simulink model "barcatet_slow_faraHold5cazuri"  (R2021a)
settings: Solver=ode8  StartTime=0.0  StopTime=inf  FixedStep=0.1  RelTol=1e-3
undefined symbols (not defined in the file): carma, distantaLimDr, distantaLimFata, distantaLimSt, motDr, motSt, V0
libraries: simulink x5, arduinolib x3, arduinosensorlib x3
settings Model: SILPILModeSetting=veronly  ExtModeTrigDuration=2  Creator=CANDRONE  LastModifiedBy=Aspire 5
settings OptimizationCC: EnhancedBackFolding=on  PassReuseOutputArgsAs=Individual arguments  ZeroExternalMemoryAtStartup=off  ZeroInternalMemoryAtStartup=off  MaxStackSize=64  OptimizeBlockOrder=speed  DifferentSizesBufferReuse=on  OptimizationCustomize=off  EfficientTunableParamExpr=on
settings DebuggingCC: ParameterTunabilityLossMsg=error
settings HardwareCC: ProdBitPerInt=16  ProdBitPerPointer=16  ProdBitPerSizeT=16  ProdBitPerPtrDiffT=16  ProdLargestAtomicFloat=None  ProdWordSize=8  ProdHWDeviceType=Atmel->AVR
settings SFSimCC: MATLABDynamicMemAlloc=off
settings RTWCC: SystemTargetFile=ert.tlc  HardwareBoard=Arduino Mega 2560  TemplateMakefile=ert_default_tmf  Toolchain=Arduino AVR
settings CodeAppCC: ForceParamTrailComments=on  IgnoreCustomStorageClasses=off  OperatorAnnotations=on  SimulinkDataObjDesc=on  SFDataObjDesc=on  InsertBlockDesc=on
settings ERTTargetCC: SupportContinuousTime=on  SupportVariableSizeSignals=on  ExtModeStaticAllocSize=2048

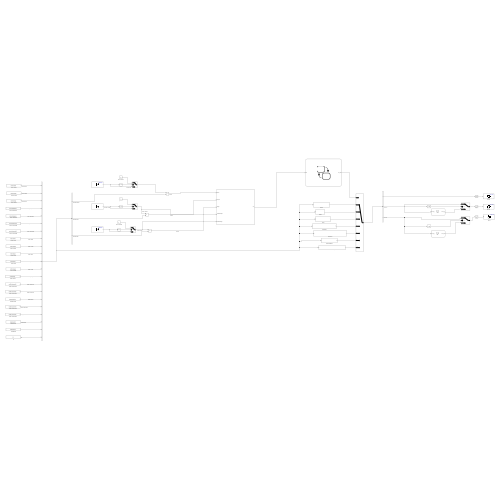
[thumbnail: Simulink's stored preview of the top-level diagram]
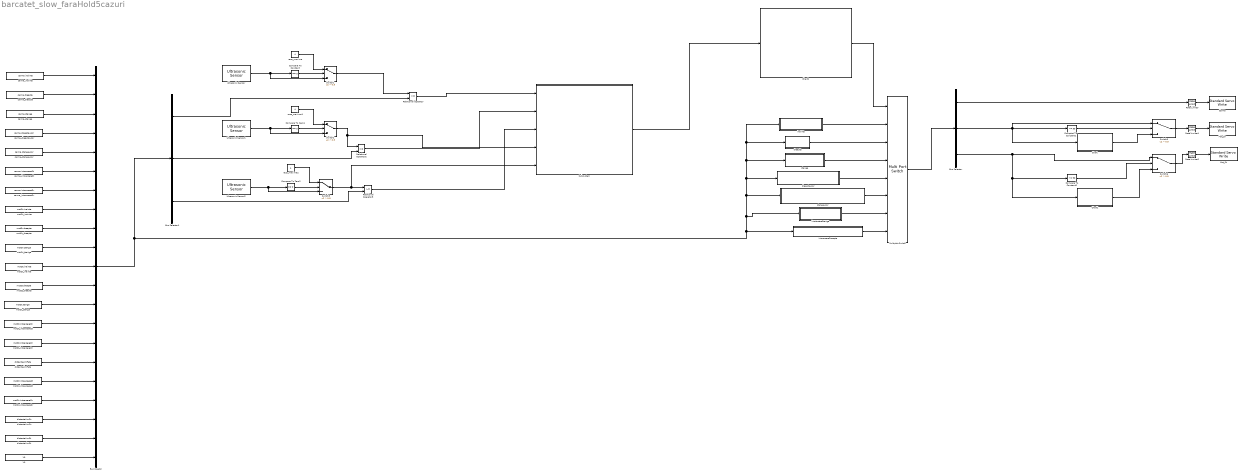
== system barcatet_slow_faraHold5cazuri ==
  Bus Creator : BusCreator  Inputs=21
  Bus Selector : BusSelector  OutputSignals=carma,mot_Dr,mot_St
  Bus Selector1 : BusSelector  OutputSignals=distantaLimFata,distantaLimDr,distantaLimSt
  Carma : arduinolib/Standard Servo Write  pinNumber=3  ServoIndex=0  blockPlatform=ARDUINO
  Chart : Stateflow chart  TreatAsAtomicUnit=on
  Chart1 : Stateflow chart  TreatAsAtomicUnit=on
  Chart2 : Stateflow chart  TreatAsAtomicUnit=on
      settings: PortSchema="{\"entries\":[{\"content\":{\"sides\":[{\"content\":{\"connectorIds\":[]},\"type\":\"ConnectorPlacement.EquallySpacedRectSide\",\"uuid\":\"b65892ab-a4a5-42cf-9574-b562b3ab09c8\"},{\"content\":{\"connectorIds\":[],\"side\":\"RIGHT\"},\"type\":\"ConnectorPlacement.EquallySpacedRectSide\",\"uuid\":\"2dcb0f11-f557-44d4-b00c-5c1b46d969f3\"},{\"content\":{\"connectorIds\":[\"In1\"],\"side\":\"TOP\"},\"type\":\"ConnectorPlacement.EquallySpacedRectSide\",\"uuid\":\"90dfae61-e3ee-4f1a-8a1b-e6404f475ac4\"},{\"content\":{\"connectorIds\":[\"Out1\"],\"side\":\"BOTTOM\"},\"type\":\"ConnectorPlacement.EquallySpacedRectSide\",\"uuid\":\"1ae09705-4430-49f5-b771-2622bfcf56ac\"}]},\"type\":\"ConnectorPlacement.EquallySpacedConnector\",\"uuid\":\"e4b1cea4-b3a8-4687-a2b3-29b89c5ba45a\"}],\"packageUris\":[\"http://schema.mathworks.com/mf0/Connector/R2020b\"],\"version\":\"1.0\"}"
  Compare To Constant : simulink/Logic and Bit Operations/Compare To Constant  relop===  const=0  OutDataTypeStr=boolean
  Compare To Constant1 : simulink/Logic and Bit Operations/Compare To Constant  relop=>=  const=90  OutDataTypeStr=boolean
  Compare To Constant2 : simulink/Logic and Bit Operations/Compare To Constant  relop=>=  const=90  OutDataTypeStr=boolean
  Compare To Zero1 : simulink/Logic and Bit Operations/Compare To Zero  relop===  OutDataTypeStr=boolean
  Compare To Zero2 : simulink/Logic and Bit Operations/Compare To Zero  relop===  OutDataTypeStr=boolean
  Inainte : Subsystem
  IntoarcereDreapta : Subsystem
  Mot_Dr : arduinolib/Standard Servo Write  pinNumber=5  ServoIndex=1  blockPlatform=ARDUINO
  Mot_St : arduinolib/Standard Servo Write  pinNumber=4  ServoIndex=2  blockPlatform=ARDUINO
  Multiport Switch : MultiPortSwitch  Inputs=7  DiagnosticForDefault=None
  Rate Limiter : RateLimiter  RisingSlewLimit=5000  FallingSlewLimit=-5000  SampleTimeMode=inherited
  Rate Limiter1 : RateLimiter  RisingSlewLimit=250  FallingSlewLimit=-250  SampleTimeMode=inherited
  Rate Limiter2 : RateLimiter  RisingSlewLimit=250  FallingSlewLimit=-250  SampleTimeMode=inherited
  Relational Operator : RelationalOperator  OutDataTypeStr=boolean  RndMeth=Simplest
  Relational Operator2 : RelationalOperator  OutDataTypeStr=boolean  RndMeth=Simplest
  Relational Operator3 : RelationalOperator  OutDataTypeStr=boolean  RndMeth=Simplest
  Subsystem : Subsystem
  Switch{1..3,5..6} (5 alike) : Switch  Criteria=u2 > Threshold  Threshold=0.5
  Ultrasonic Sensor : arduinosensorlib/Ultrasonic Sensor  NumSignalPins=2  TrigPin=6  EchoPin=12  SignalPin=3  SampleTime_=0.1  blockPlatform=ARDUINO
      settings: SourceProductBaseCode=ARDUINO
  Ultrasonic Sensor1 : arduinosensorlib/Ultrasonic Sensor  NumSignalPins=2  TrigPin=10  EchoPin=2  SignalPin=3  SampleTime_=0.1  blockPlatform=ARDUINO
      settings: SourceProductBaseCode=ARDUINO
  Ultrasonic Sensor2 : arduinosensorlib/Ultrasonic Sensor  NumSignalPins=2  TrigPin=11  EchoPin=9  SignalPin=3  SampleTime_=0.1  blockPlatform=ARDUINO
      settings: SourceProductBaseCode=ARDUINO
  V0 : Constant  Value=V0
  carma_dreapta : Constant  Value=carma.dreapta
  carma_dreaptausor : Constant  Value=carma.dreaptausor
  carma_inainte : Constant  Value=carma.inainte
  carma_intoarcereDr : Constant  Value=carma.intoarcereDr
  carma_intoarcereSt : Constant  Value=carma.intoarcereSt
  carma_stanga : Constant  Value=carma.stanga
  carma_stangausor : Constant  Value=carma.stangausor
  distantaLimDr : Constant  Value=distantaLimDr
  distantaLimFata : Constant  Value=distantaLimFata
  distantaLimSt : Constant  Value=distantaLimSt
  dreapta : Subsystem
  dreaptausor : Subsystem
  intoarcereStanga : Subsystem
  motDr_dreapta : Constant  Value=motDr.dreapta
  motDr_inainte : Constant  Value=motDr.inainte
  motDr_intoarcereDr : Constant  Value=motDr.intoarcereDr
  motDr_intoarcereSt : Constant  Value=motDr.intoarcereSt
  motDr_stanga : Constant  Value=motDr.stanga
  motSt_dreapta : Constant  Value=motSt.dreapta
  motSt_inainte : Constant  Value=motSt.inainte
  motSt_intoarcereDr : Constant  Value=motSt.intoarcereDr
  motSt_intoarcereSt : Constant  Value=motSt.intoarcereSt
  motSt_stanga : Constant  Value=motSt.stanga
  raza_maxima : Constant  Value=4
  raza_maxima1 : Constant  Value=4
  raza_maxima2 : Constant  Value=4
  stanga : Subsystem
  stangausor : Subsystem
  wires:
  Bus Selector1/1 -> Relational Operator/2  "<distantaLimFata>"
  Bus Selector/1 -> Rate Limiter/1  "<carma>"
  Bus Selector/2 -> Chart/1(amot_Dr_), Switch5/1, Compare To Constant1/1  "<mot_Dr>"
  Ultrasonic Sensor1/1 -> Switch2/3, Compare To Zero1/1  "Semnal_dreapta"
  Compare To Zero1/1 -> Switch2/2
  Ultrasonic Sensor/1 -> Switch1/3, Compare To Constant/1  "Semnal_fata"
  Compare To Constant/1 -> Switch1/2
  raza_maxima/1 -> Switch1/1
  Switch1/1 -> Relational Operator/1
  raza_maxima1/1 -> Switch2/1
  Ultrasonic Sensor2/1 -> Switch3/3, Compare To Zero2/1  "semnal_stanga"
  raza_maxima2/1 -> Switch3/1
  Compare To Zero2/1 -> Switch3/2
  Switch2/1 -> Subsystem/4(DistantaDreapta), Relational Operator2/1  "semnal_dreapta"
  Switch3/1 -> Subsystem/5(DistantaStanga), Relational Operator3/1  "semnal_stanga"
  Rate Limiter/1 -> Carma/1
  Rate Limiter1/1 -> Mot_Dr/1
  Rate Limiter2/1 -> Mot_St/1
  Bus Selector/3 -> Chart1/1(amot_St_), Compare To Constant2/1, Switch6/1  "<mot_St>"
  Compare To Constant1/1 -> Switch5/2
  Switch5/1 -> Rate Limiter1/1
  Chart/1(mot_Out) -> Switch5/3
  Compare To Constant2/1 -> Switch6/2
  Switch6/1 -> Rate Limiter2/1
  Chart1/1(mot_Out) -> Switch6/3
  Multiport Switch/1 -> Bus Selector/1
  carma_inainte/1 -> Bus Creator/1  "carma_inainte"
  carma_dreapta/1 -> Bus Creator/2  "carma_dreapta"
  carma_stanga/1 -> Bus Creator/3  "carma_stanga"
  carma_dreaptausor/1 -> Bus Creator/4  "carma_dreaptausor"
  carma_stangausor/1 -> Bus Creator/5  "carma_stangausor"
  carma_intoarcereSt/1 -> Bus Creator/6  "carma_intoarcereSt"
  carma_intoarcereDr/1 -> Bus Creator/7  "carma_intoarcereDr"
  motDr_dreapta/1 -> Bus Creator/9  "motDr_dreapta"
  motDr_stanga/1 -> Bus Creator/10  "motDr_stanga"
  motDr_inainte/1 -> Bus Creator/8  "motDr_inainte"
  motSt_inainte/1 -> Bus Creator/11  "motSt_inainte"
  motSt_dreapta/1 -> Bus Creator/12  "motSt_dreapta"
  motSt_stanga/1 -> Bus Creator/13  "motSt_stanga"
  motSt_intoarcereSt/1 -> Bus Creator/14  "motSt_intoarcereSt"
  motSt_intoarcereDr/1 -> Bus Creator/15  "motSt_intoarcereDr"
  distantaLimFata/1 -> Bus Creator/16  "distantaLimFata"
  Inainte/1(Out1) -> Multiport Switch/2
  dreapta/1(Out1) -> Multiport Switch/3
  stanga/1(Out1) -> Multiport Switch/4
  dreaptausor/1(Out1) -> Multiport Switch/5
  stangausor/1(Out1) -> Multiport Switch/6
  Bus Creator/1 -> Bus Selector1/1, Inainte/1(In1), dreapta/1(In1), stanga/1(In1), dreaptausor/1(In1), stangausor/1(In1), intoarcereStanga/1(In1), IntoarcereDreapta/1(In1)
  motDr_intoarcereSt/1 -> Bus Creator/17  "motDr_intoarcereSt"
  motDr_intoarcereDr/1 -> Bus Creator/18  "motDr_intoarcereDr"
  intoarcereStanga/1(Out1) -> Multiport Switch/7
  IntoarcereDreapta/1(Out1) -> Multiport Switch/8
  distantaLimDr/1 -> Bus Creator/19  "distantaLimDr"
  distantaLimSt/1 -> Bus Creator/20  "distantaLimSt"
  Bus Selector1/2 -> Relational Operator2/2  "<distantaLimDr>"
  Bus Selector1/3 -> Relational Operator3/2  "<distantaLimSt>"
  Relational Operator/1 -> Subsystem/1(Inainte)  "Inainte"
  Relational Operator2/1 -> Subsystem/2(Dreapta)  "Dreapta"
  Relational Operator3/1 -> Subsystem/3(Stanga)  "Stanga"
  Subsystem/1(caz) -> Chart2/1(caz)
  Chart2/1(caz_out) -> Multiport Switch/1
  V0/1 -> Bus Creator/21  "V0"

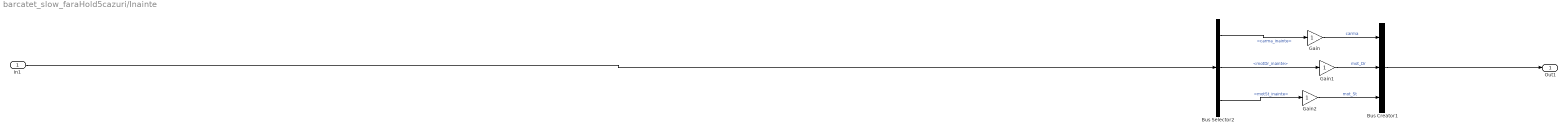
== system barcatet_slow_faraHold5cazuri/Inainte ==
  In1 : Inport
  Bus Creator1 : BusCreator  Inputs=3
  Bus Selector2 : BusSelector  OutputSignals=carma_inainte,motDr_inainte,motSt_inainte
  Gain : Gain
  Gain1 : Gain
  Gain2 : Gain
  Out1 : Outport
  wires:
  Gain2/1 -> Bus Creator1/3  "mot_St"
  Bus Selector2/3 -> Gain2/1  "<motSt_inainte>"
  Bus Selector2/1 -> Gain/1  "<carma_inainte>"
  Gain1/1 -> Bus Creator1/2  "mot_Dr"
  Bus Selector2/2 -> Gain1/1  "<motDr_inainte>"
  Gain/1 -> Bus Creator1/1  "carma"
  Bus Creator1/1 -> Out1/1
  In1/1 -> Bus Selector2/1

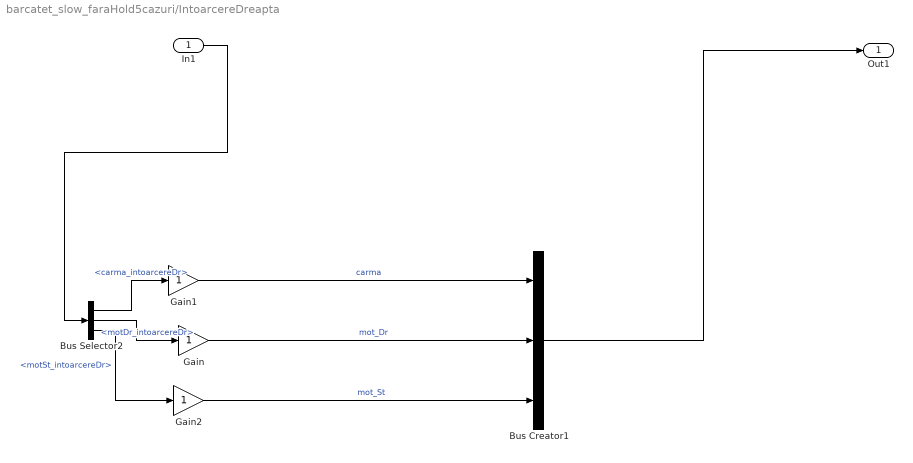
== system barcatet_slow_faraHold5cazuri/IntoarcereDreapta ==
  In1 : Inport
  Bus Creator1 : BusCreator  Inputs=3
  Bus Selector2 : BusSelector  OutputSignals=carma_intoarcereDr,motDr_intoarcereDr,motSt_intoarcereDr
  Gain : Gain
  Gain1 : Gain
  Gain2 : Gain
  Out1 : Outport
  wires:
  Gain1/1 -> Bus Creator1/1  "carma"
  Gain/1 -> Bus Creator1/2  "mot_Dr"
  Bus Selector2/1 -> Gain1/1  "<carma_intoarcereDr>"
  Bus Selector2/2 -> Gain/1  "<motDr_intoarcereDr>"
  Bus Selector2/3 -> Gain2/1  "<motSt_intoarcereDr>"
  Gain2/1 -> Bus Creator1/3  "mot_St"
  In1/1 -> Bus Selector2/1
  Bus Creator1/1 -> Out1/1

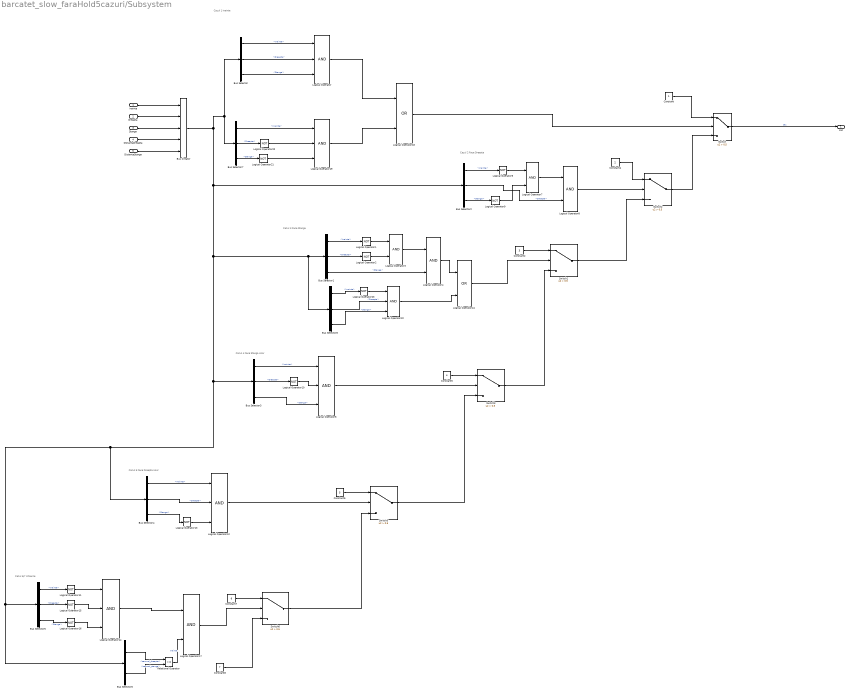
== system barcatet_slow_faraHold5cazuri/Subsystem ==
  note: Cazul 3 Face Stanga
  note: Cazul 2 Face Dreapta
  note: Cazul 1 Inainte
  note: Cazul 4 Face Stanga Usor
  note: Cazul 5 Face Dreapta Usor
  note: Cazul 6/7 Intoarce
  Inainte : Inport
  Dreapta : Inport  Port=2
  Stanga : Inport  Port=3
  DistantaDreapta : Inport  Port=4
  DistantaStanga : Inport  Port=5
  Bus Creator : BusCreator  Inputs=5
  Bus Selector{,1..5,7..8} (8 alike) : BusSelector  OutputSignals=Inainte,Dreapta,Stanga
  Bus Selector6 : BusSelector  OutputSignals=semnal_dreapta,semnal_stanga
  Constant : Constant  OutDataTypeStr=double
  Constant2 : Constant  Value=3
  Constant4 : Constant  Value=2
  Constant5 : Constant  Value=4
  Constant6 : Constant  Value=5
  Constant7 : Constant  Value=6
  Constant8 : Constant  Value=7
  Logical Operator{,6,12,14,19,22} (6 alike) : Logic  Inputs=3  AllPortsSameDT=off  OutDataTypeStr=boolean
  Logical Operator{1..2,5,9..11,13,15..16,20..21,23} (12 alike) : Logic  Operator=NOT  AllPortsSameDT=off  OutDataTypeStr=boolean
  Logical Operator{3..4,7..8,17} (5 alike) : Logic  AllPortsSameDT=off  OutDataTypeStr=boolean
  Logical Operator18 : Logic  Operator=OR  AllPortsSameDT=off  OutDataTypeStr=boolean
  Logical Operator24 : Logic  Operator=OR  AllPortsSameDT=off  OutDataTypeStr=boolean
  Relational Operator : RelationalOperator  OutDataTypeStr=boolean  RndMeth=Simplest
  Switch{,1..3,5..6} (6 alike) : Switch  Criteria=u2 > Threshold  Threshold=0.5  OutDataTypeStr=double
  caz : Outport
  wires:
  Switch2/1 -> Switch/3
  Logical Operator18/1 -> Switch/2
  Constant/1 -> Switch/1
  Inainte/1 -> Bus Creator/1
  Dreapta/1 -> Bus Creator/2
  Stanga/1 -> Bus Creator/3
  Switch/1 -> caz/1  "caz"
  Bus Selector/1 -> Logical Operator/1  "<Inainte>"
  Bus Selector/2 -> Logical Operator/2  "<Dreapta>"
  Bus Selector/3 -> Logical Operator/3  "<Stanga>"
  Constant2/1 -> Switch1/1
  Bus Selector1/1 -> Logical Operator1/1  "<Inainte>"
  Bus Selector1/2 -> Logical Operator2/1  "<Dreapta>"
  Bus Selector1/3 -> Logical Operator4/2  "<Stanga>"
  Logical Operator1/1 -> Logical Operator3/1
  Logical Operator2/1 -> Logical Operator3/2
  Logical Operator3/1 -> Logical Operator4/1
  Logical Operator24/1 -> Switch1/2
  Logical Operator8/1 -> Switch2/2
  Bus Selector2/2 -> Logical Operator8/2  "<Dreapta>"
  Constant4/1 -> Switch2/1
  Bus Selector2/3 -> Logical Operator9/1  "<Stanga>"
  Bus Selector2/1 -> Logical Operator5/1  "<Inainte>"
  Logical Operator5/1 -> Logical Operator7/1
  Logical Operator7/1 -> Logical Operator8/1
  Logical Operator9/1 -> Logical Operator7/2
  Switch1/1 -> Switch2/3
  Logical Operator6/1 -> Switch3/2
  Bus Selector3/2 -> Logical Operator10/1  "<Dreapta>"
  Bus Selector3/3 -> Logical Operator6/3  "<Stanga>"
  Bus Selector3/1 -> Logical Operator6/1  "<Inainte>"
  Logical Operator10/1 -> Logical Operator6/2
  Constant5/1 -> Switch3/1
  Switch3/1 -> Switch1/3
  Switch5/1 -> Switch3/3
  Logical Operator12/1 -> Switch5/2
  Switch6/1 -> Switch5/3
  Bus Selector4/2 -> Logical Operator12/2  "<Dreapta>"
  Constant6/1 -> Switch5/1
  Bus Selector4/3 -> Logical Operator13/1  "<Stanga>"
  Bus Selector4/1 -> Logical Operator12/1  "<Inainte>"
  Logical Operator13/1 -> Logical Operator12/3
  Logical Operator14/1 -> Logical Operator17/1
  Constant8/1 -> Switch6/3
  Bus Creator/1 -> Bus Selector7/1, Bus Selector/1, Bus Selector2/1, Bus Selector6/1, Bus Selector5/1, Bus Selector4/1, Bus Selector3/1, Bus Selector8/1, Bus Selector1/1
  Constant7/1 -> Switch6/1
  Bus Selector5/1 -> Logical Operator11/1  "<Inainte>"
  DistantaDreapta/1 -> Bus Creator/4
  DistantaStanga/1 -> Bus Creator/5
  Logical Operator11/1 -> Logical Operator14/1
  Bus Selector5/2 -> Logical Operator15/1  "<Dreapta>"
  Bus Selector5/3 -> Logical Operator16/1  "<Stanga>"
  Logical Operator15/1 -> Logical Operator14/2
  Logical Operator16/1 -> Logical Operator14/3
  Bus Selector6/1 -> Relational Operator/1  "<semnal_dreapta>"
  Bus Selector6/2 -> Relational Operator/2  "<semnal_stanga>"
  Relational Operator/1 -> Logical Operator17/2  "Inainte"
  Logical Operator17/1 -> Switch6/2
  Logical Operator/1 -> Logical Operator18/1
  Bus Selector7/1 -> Logical Operator19/1  "<Inainte>"
  Bus Selector7/2 -> Logical Operator20/1  "<Dreapta>"
  Logical Operator20/1 -> Logical Operator19/2
  Logical Operator21/1 -> Logical Operator19/3
  Bus Selector7/3 -> Logical Operator21/1  "<Stanga>"
  Logical Operator19/1 -> Logical Operator18/2
  Bus Selector8/1 -> Logical Operator23/1  "<Inainte>"
  Logical Operator23/1 -> Logical Operator22/1
  Bus Selector8/2 -> Logical Operator22/2  "<Dreapta>"
  Bus Selector8/3 -> Logical Operator22/3  "<Stanga>"
  Logical Operator22/1 -> Logical Operator24/2
  Logical Operator4/1 -> Logical Operator24/1

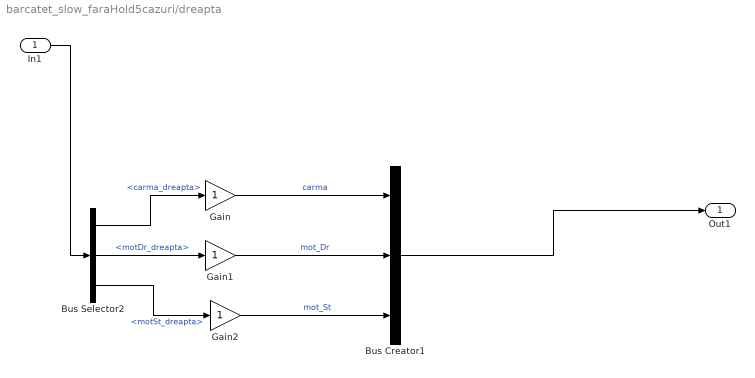
== system barcatet_slow_faraHold5cazuri/dreapta ==
  In1 : Inport
  Bus Creator1 : BusCreator  Inputs=3
  Bus Selector2 : BusSelector  OutputSignals=carma_dreapta,motDr_dreapta,motSt_dreapta
  Gain : Gain
  Gain1 : Gain
  Gain2 : Gain
  Out1 : Outport
  wires:
  Bus Selector2/1 -> Gain/1  "<carma_dreapta>"
  Bus Selector2/2 -> Gain1/1  "<motDr_dreapta>"
  Gain/1 -> Bus Creator1/1  "carma"
  Gain1/1 -> Bus Creator1/2  "mot_Dr"
  Gain2/1 -> Bus Creator1/3  "mot_St"
  In1/1 -> Bus Selector2/1
  Bus Selector2/3 -> Gain2/1  "<motSt_dreapta>"
  Bus Creator1/1 -> Out1/1

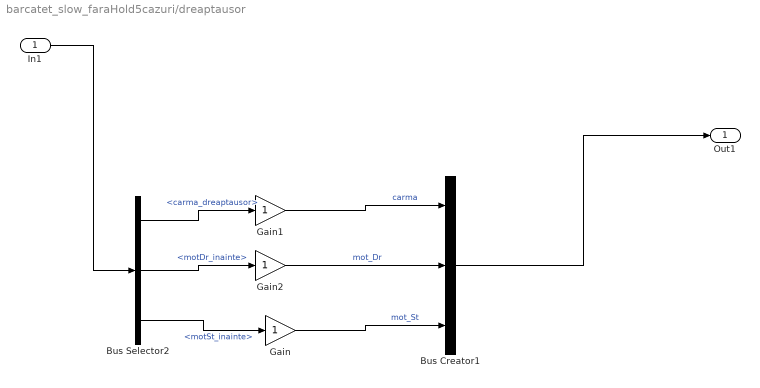
== system barcatet_slow_faraHold5cazuri/dreaptausor ==
  In1 : Inport
  Bus Creator1 : BusCreator  Inputs=3
  Bus Selector2 : BusSelector  OutputSignals=carma_dreaptausor,motDr_inainte,motSt_inainte
  Gain : Gain
  Gain1 : Gain
  Gain2 : Gain
  Out1 : Outport
  wires:
  Gain/1 -> Bus Creator1/3  "mot_St"
  Gain2/1 -> Bus Creator1/2  "mot_Dr"
  Gain1/1 -> Bus Creator1/1  "carma"
  Bus Selector2/3 -> Gain/1  "<motSt_inainte>"
  Bus Creator1/1 -> Out1/1
  In1/1 -> Bus Selector2/1
  Bus Selector2/2 -> Gain2/1  "<motDr_inainte>"
  Bus Selector2/1 -> Gain1/1  "<carma_dreaptausor>"

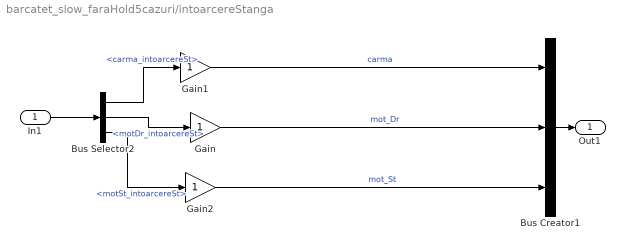
== system barcatet_slow_faraHold5cazuri/intoarcereStanga ==
  In1 : Inport
  Bus Creator1 : BusCreator  Inputs=3
  Bus Selector2 : BusSelector  OutputSignals=carma_intoarcereSt,motDr_intoarcereSt,motSt_intoarcereSt
  Gain : Gain
  Gain1 : Gain
  Gain2 : Gain
  Out1 : Outport
  wires:
  Gain1/1 -> Bus Creator1/1  "carma"
  Bus Selector2/3 -> Gain2/1  "<motSt_intoarcereSt>"
  Bus Selector2/2 -> Gain/1  "<motDr_intoarcereSt>"
  Gain/1 -> Bus Creator1/2  "mot_Dr"
  Bus Creator1/1 -> Out1/1
  Bus Selector2/1 -> Gain1/1  "<carma_intoarcereSt>"
  Gain2/1 -> Bus Creator1/3  "mot_St"
  In1/1 -> Bus Selector2/1

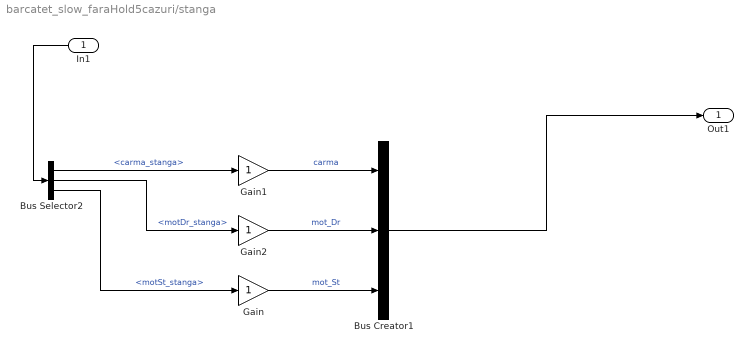
== system barcatet_slow_faraHold5cazuri/stanga ==
  In1 : Inport
  Bus Creator1 : BusCreator  Inputs=3
  Bus Selector2 : BusSelector  OutputSignals=carma_stanga,motDr_stanga,motSt_stanga
  Gain : Gain
  Gain1 : Gain
  Gain2 : Gain
  Out1 : Outport
  wires:
  Bus Selector2/3 -> Gain/1  "<motSt_stanga>"
  Bus Selector2/1 -> Gain1/1  "<carma_stanga>"
  Bus Creator1/1 -> Out1/1
  Gain/1 -> Bus Creator1/3  "mot_St"
  Gain2/1 -> Bus Creator1/2  "mot_Dr"
  Bus Selector2/2 -> Gain2/1  "<motDr_stanga>"
  Gain1/1 -> Bus Creator1/1  "carma"
  In1/1 -> Bus Selector2/1

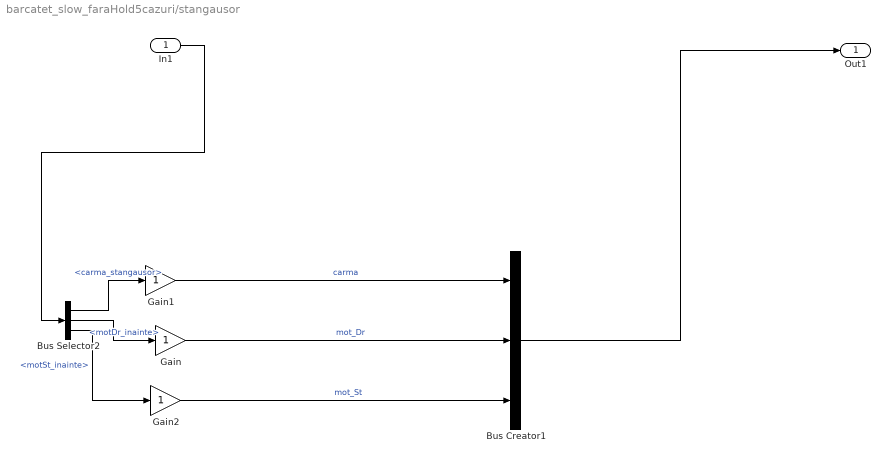
== system barcatet_slow_faraHold5cazuri/stangausor ==
  In1 : Inport
  Bus Creator1 : BusCreator  Inputs=3
  Bus Selector2 : BusSelector  OutputSignals=carma_stangausor,motDr_inainte,motSt_inainte
  Gain : Gain
  Gain1 : Gain
  Gain2 : Gain
  Out1 : Outport
  wires:
  Gain1/1 -> Bus Creator1/1  "carma"
  Gain/1 -> Bus Creator1/2  "mot_Dr"
  Bus Selector2/1 -> Gain1/1  "<carma_stangausor>"
  Bus Selector2/2 -> Gain/1  "<motDr_inainte>"
  Bus Selector2/3 -> Gain2/1  "<motSt_inainte>"
  Gain2/1 -> Bus Creator1/3  "mot_St"
  In1/1 -> Bus Selector2/1
  Bus Creator1/1 -> Out1/1

== stateflow chart barcatet_slow_faraHold5cazuri/Chart1 ==
  state reverse_2
    mot_Out = 60;
  state reverse_1
    mot_Out = 90;
  state Reverse_e_activ
    entry:
    mot_Out = 90;
  state reverse_3
    mot_Out = 60;
  reverse_2 -> Reverse_e_activ : [amot_St_ >= 90]
  reverse_1 -> reverse_2 : [after(200,msec)]
  (default) -> Reverse_e_activ
  reverse_3 -> reverse_1 : after(200,msec)
  Reverse_e_activ -> reverse_3 : [amot_St_ < 90]
  data: mot_Out output; amot_St_ input

== stateflow chart barcatet_slow_faraHold5cazuri/Chart2 ==
  state default1
    entry:
    caz_out = caz;
    caz_intern = caz;
  state default
    entry:
    caz_out = caz;
    caz_intern = caz;
  state default2
    entry:
    caz_out = caz_intern;
  (default) -> default
  default -> (junction 12) : [hasChanged(caz)]
  (junction 12) -> default1 [order 2] : [caz ~=1]
  (junction 12) -> default [order 1] : [caz ==1]
  default1 -> default2 : [after(10,msec)]
  default2 -> default : [after(0.5,sec)]
  data: caz input double; caz_out output double; caz_intern local

== stateflow chart barcatet_slow_faraHold5cazuri/Chart ==
  state reverse_2
    mot_Out = 60;
  state reverse_1
    mot_Out = 90;
  state Reverse_e_activ
    entry:
    mot_Out = 90;
  state reverse_3
    mot_Out = 60;
  reverse_2 -> Reverse_e_activ : [amot_Dr_ >= 90]
  reverse_1 -> reverse_2 : [after(200,msec)]
  (default) -> Reverse_e_activ
  reverse_3 -> reverse_1 : after(200,msec)
  Reverse_e_activ -> reverse_3 : [amot_Dr_ < 90]
  data: mot_Out output; amot_Dr_ input
